simulink model "Q4_1"  (R2021a)
settings: Solver=VariableStepAuto  StartTime=0.0  StopTime=10.0  RelTol=1e-3
settings Model: OrderedModelArguments=off  Creator=sachi  LastModifiedBy=sachi

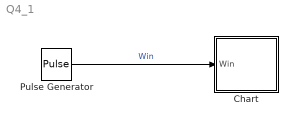
== system Q4_1 ==
  Chart : Stateflow chart  TreatAsAtomicUnit=on
  Pulse Generator : DiscretePulseGenerator  PulseType=Time based  Period=10  PulseWidth=5
  wires:
  Pulse Generator/1 -> Chart/1(Win)  "Win"

== stateflow chart Q4_1/Chart ==
  state Init
    exit:
    l_R = l_R0;
    L_1 = l_10;
    l_2 = l_20;
    l_3 = l_30;
    thetad = thetad0;
    uc = uc0;
  state Dyns
    during:
    l_R_dot = 1/(pi*(r0_R+l_R)^2)*(Win - pi*r1^2*sqrt(2*g*(l_R+L1)) - pi*r1^2*sqrt(2*g*(l_R+L1)));
    l_1_dot = 1/(pi * r1^2)*(pi*rt1^2*sqrt(2*g*(l_R+L1)) - betaT*(1-tau)*(rho*g*(l_1-l_2)));
    l_2_dot = 1/(pi * r2^2)*(pi*rt2^2*sqrt(2*g*(l_R+L2)) + betaT*(1-tau)*(rho*g*(l_1-l_2))- beta3*(rho*g*(l_2-l_3)));
    l_3_dot = 1/(pi * r3^2)*(beta3*(rho*g*(l_2-l_3)) - pi*rtOut^2*sqrt(2*g*(l_3+Lout)));
    thetad_dot = 1/J*(R2/R1)^2*eps*betaT*tau*(1-tau)*(rho*g*(l_1-l_2))^2*thetad + 1/R*(Kr*uc + Kr^2*thetad);
    uc_dot = -1/C*R * (uc + Kr*thetad);
  (default) -> (junction 12)
  Init -> Dyns
  data: Win input
